simulink model "ModelEx1"  (R2018b)
settings: Solver=ode4  StartTime=0.0  StopTime=10.0  FixedStep=0.01  RelTol=1e-3
values from neighbouring files (symbols this model uses):
  alfa = WPC(i)    [ScriptEx1.m]
  L = WPC(i)    [ScriptEx1.m]
  x0 = 1.5    [ScriptEx1.m]    (also in ScriptEx4.m = x0-W(x1)/Wprim(x1))
settings Model: Creator=Joanna  LastModifiedBy=Joanna

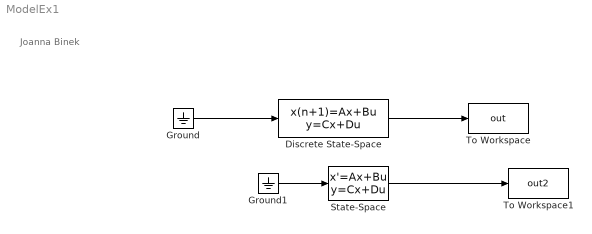
== system ModelEx1 ==
  note: Joanna Binek
  Discrete State-Space : DiscreteStateSpace  A=L  B=0  D=0  InitialCondition=x0
  Ground : Ground
  Ground1 : Ground
  State-Space : StateSpace  A=alfa  B=0  D=0  InitialCondition=x0
  To Workspace : ToWorkspace  VariableName=out  SampleTime=-1
  To Workspace1 : ToWorkspace  VariableName=out2  SampleTime=-1
  wires:
  Ground/1 -> Discrete State-Space/1
  Discrete State-Space/1 -> To Workspace/1
  Ground1/1 -> State-Space/1
  State-Space/1 -> To Workspace1/1
